simulink model "simulation"  (R2021a)
settings: Solver=VariableStepAuto  StartTime=0.0  StopTime=10  RelTol=1e-3
model workspace (MAT data in the model file):
  D = 0.403776507668
  Dtheta = 0.380153322744
  Sig = Simulink.Signal
  Sig.DataType = 'auto'
  Sig.Dimensions = -1
  Sig.DimensionsMode = 'auto'
  Sig.Complexity = 'auto'
  Sig.SampleTime = -1
  Sig.SamplingMode = 'auto'
  T = 0.218447386965
  Ttheta = 0.106008422232
libraries: SignalEditorBlockLib x1
settings Model: Creator=Marvin  LastModifiedBy=Marvin

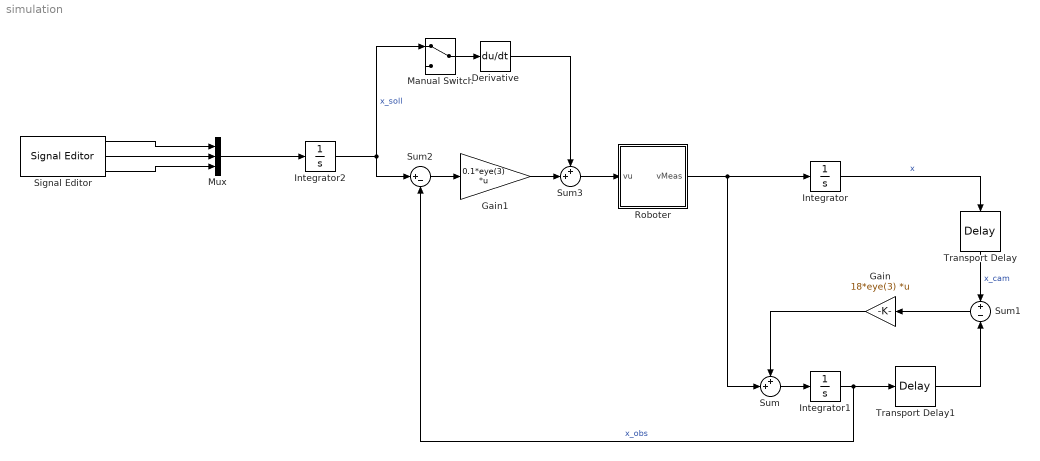
== system simulation ==
  Derivative : Derivative
  Gain : Gain  Gain=18*eye(3)  Multiplication=Matrix(K*u)
  Gain1 : Gain  Gain=0.1*eye(3)  Multiplication=Matrix(K*u)
  Integrator : Integrator
  Integrator1 : Integrator
  Integrator2 : Integrator
  Manual Switch : ManualSwitch
  Mux : Mux  Inputs=3
  Roboter : Subsystem
  Signal Editor : SignalEditorBlockLib/Signal Editor  FileName=untitled.mat  ActiveScenario=SprungX  ActiveSignal=x  IsBus=off  OutputBusObjectStr=Bus: BusObject  SampleTime=0  Interpolate=off  ZeroCross=off  OutputAfterFinalValue=Setting to zero  Unit=inherit  PreserveSignalName=on
  Sum : Sum  Inputs=++|
  Sum1 : Sum  Inputs=+|-
  Sum2 : Sum  Inputs=|+-
  Sum3 : Sum  Inputs=++|
  Transport Delay : TransportDelay  DelayTime=0.04
  Transport Delay1 : TransportDelay  DelayTime=0.14
  wires:
  Integrator/1 -> Transport Delay/1  "x"
  Roboter/1(vMeas) -> Sum/2, Integrator/1
  Sum/1 -> Integrator1/1
  Integrator1/1 -> Sum2/2, Transport Delay1/1  "x_obs"
  Transport Delay1/1 -> Sum1/2
  Transport Delay/1 -> Sum1/1  "x_cam"
  Sum1/1 -> Gain/1
  Gain/1 -> Sum/1
  Signal Editor/2 -> Mux/2
  Signal Editor/3 -> Mux/3
  Sum2/1 -> Gain1/1
  Mux/1 -> Integrator2/1
  Signal Editor/1 -> Mux/1
  Gain1/1 -> Sum3/2
  Integrator2/1 -> Manual Switch/1, Sum2/1  "x_soll"
  Sum3/1 -> Roboter/1(vu)
  Derivative/1 -> Sum3/1
  Manual Switch/1 -> Derivative/1

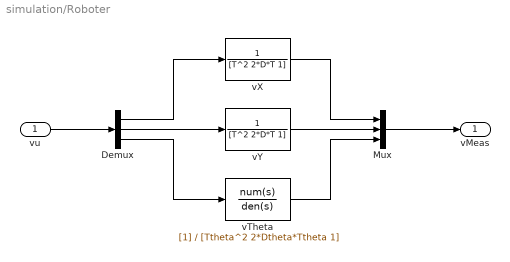
== system simulation/Roboter ==
  vu : Inport
  Demux : Demux  Outputs=3
  Mux : Mux  Inputs=3
  vTheta : TransferFcn  Denominator=[Ttheta^2 2*Dtheta*Ttheta 1]
  vX : TransferFcn  Denominator=[T^2 2*D*T 1]
  vY : TransferFcn  Denominator=[T^2 2*D*T 1]
  vMeas : Outport
  wires:
  vY/1 -> Mux/2
  Demux/1 -> vX/1
  Mux/1 -> vMeas/1
  vX/1 -> Mux/1
  Demux/2 -> vY/1
  vTheta/1 -> Mux/3
  Demux/3 -> vTheta/1
  vu/1 -> Demux/1
